simulink model "dual500MHzPFB"  (Simulink 6.2)
settings: Solver=ode45  StartTime=0.0  StopTime=10000  RelTol=1e-3
libraries: xbsIndex_r3 x2070, casper_library x180, xps_library x12, gtkWave x5, gavrt_library x1
(part 1 of 20)
settings Model: LastModifiedBy=Glenn
settings DebuggingCC: SolverPrmCheckMsg=warning

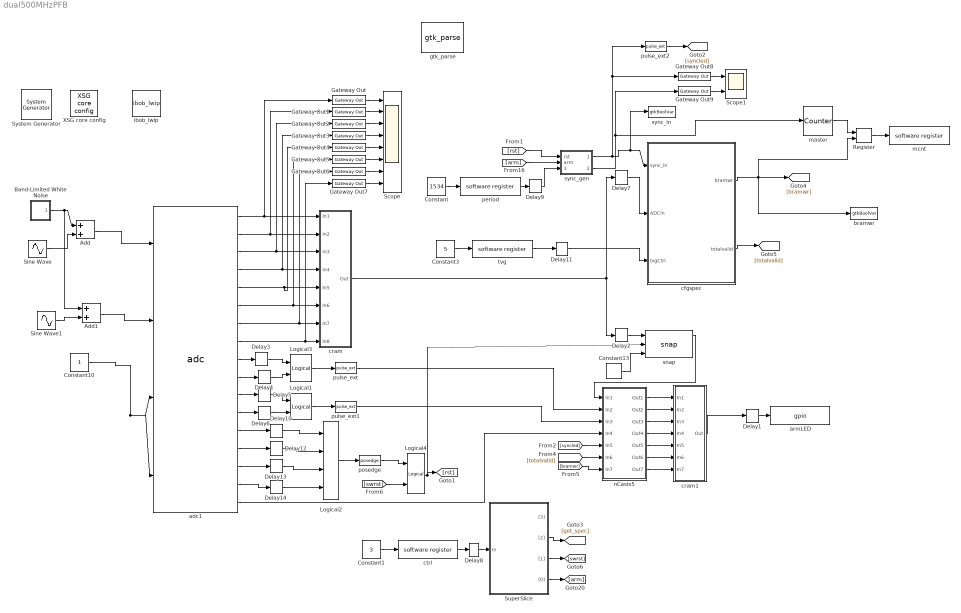
== system dual500MHzPFB ==
  " System Generator" : xbsIndex_r3/ System Generator  Tag=genX  xilinxfamily=Virtex2P  part=xc2vp50  speed=-7  package=ff1152  synthesis_tool=XST  directory=C:/casper_work/scratch/newspec/dual500MHzPFB/sysgen  testbench=off  simulink_period=1  sysclk_period=3.9063  incr_netlist=off  trim_vbits=Everywhere in SubSystem  dbl_ovrd=According to Block Masks  core_generation=According to Block Masks  run_coregen=off  deprecated_control=off  eval_field=0
      settings: AttributesFormatString=System\nGenerator
  Add : Sum  OutScaling=2^-10
  Add1 : Sum  OutScaling=2^-10
  Band-Limited White Noise : Subsystem  AncestorBlock=simulink/Sources/Band-Limited White Noise  mask(Band-Limited White Noise.){Cov=0, Ts=0.25, seed=[23341], VectorParams1D=on}
      mask prompts: Cov "Noise power:"; Ts "Sample time:"; VectorParams1D "Interpret vector parameters as 1-D"
      mask help: The Band-Limited White Noise block generates normally distributed random numbers that are suitable for use in continuous or hybrid systems.
      mask init:
      | if any(Cov < 0),
      | 	error('The ''Noise power'' must be positive. '),
      | end;
      | 
      | r = [-0.4326
      |    -1.6656
      |     0.1253
      |     0.2877
      |    -1.1465
      |     1.1909
      |     1.1892
      |    -0.0376
      |     0.3273
      |     0.1746
      |    -0.1867
      |     0.7258]';
      | 
      | r2 = [r(1),r;r,r(12)]; 
      | t =[1:13;1:13]; 
      | 
      | if any(Ts==-1), 
      | 	error('Sample time (-1) is set to be back-inherited from the block(s) it drives. You should explicitly specify the sample time of the source block. '), 
      | end;
      | set_param([gcb '/White Noise'],'VectorParams1D',VectorParams1D);
      mask Help: Implemented using white noise into Zero-Order Hold block. The seed and power can be vectors of the same length to produce a vector of white noise sources. For faster simulation, set sample time to the highest value possible but in accordance with the fastest dynamics of system.
      mask Display: plot(t(:),r2(:))
  Constant : Constant  Value=1534
  Constant1 : Constant  Value=3
  Constant10 : Constant
  Constant13 : xbsIndex_r3/Constant  const=1  equ=P=C  arith_type=Boolean  n_bits=8  bin_pt=0  opselect=C  inp2=PCIN>>17  opr=+  inp1=P  carry=CIN  iostate=0  explicit_period=on  period=1  dbl_ovrd=off
  Constant3 : Constant  Value=5
  Delay{1,3..6} (5 alike) : xbsIndex_r3/Delay  latency=4  reg_retiming=on  explicit_period=off  period=1  en=off  accept_only_valid=off  init_zero=on  dbl_ovrd=off  show_param=off
      settings: xl_area=[0, 0, 0, 0, 0, 0, 0]
  Delay{10,12..14} (4 alike) : xbsIndex_r3/Delay  latency=1  reg_retiming=on  explicit_period=off  period=1  en=off  accept_only_valid=off  init_zero=on  dbl_ovrd=off  show_param=off
      settings: xl_area=[0, 0, 0, 0, 0, 0, 0]
  Delay11 : xbsIndex_r3/Delay  latency=2  reg_retiming=on  explicit_period=off  period=1  en=off  accept_only_valid=off  init_zero=on  dbl_ovrd=off  show_param=off
      settings: xl_area=[0, 0, 0, 0, 0, 0, 0]
  Delay2 : xbsIndex_r3/Delay  latency=3  reg_retiming=on  explicit_period=off  period=1  en=off  accept_only_valid=off  init_zero=on  dbl_ovrd=off  show_param=off
      settings: xl_area=[0, 0, 0, 0, 0, 0, 0]
  Delay7 : xbsIndex_r3/Delay  latency=2  reg_retiming=on  explicit_period=off  period=1  en=off  accept_only_valid=off  init_zero=on  dbl_ovrd=off  show_param=off
      settings: xl_area=[0, 0, 0, 0, 0, 0, 0]
  Delay8 : xbsIndex_r3/Delay  latency=3  reg_retiming=on  explicit_period=off  period=1  en=off  accept_only_valid=off  init_zero=on  dbl_ovrd=off  show_param=off
      settings: xl_area=[0, 0, 0, 0, 0, 0, 0]
  Delay9 : xbsIndex_r3/Delay  latency=2  reg_retiming=on  explicit_period=off  period=1  en=off  accept_only_valid=off  init_zero=on  dbl_ovrd=off  show_param=off
      settings: xl_area=[0, 0, 0, 0, 0, 0, 0]
  Gateway Out{,1..9} (10 alike) : xbsIndex_r3/Gateway Out  output_type=Double  nbits=8  bin_pt=6  arith_type=Boolean  quantization=Truncate  overflow=Wrap  hdl_port=on  timing_constraint=None  locs_specified=off  LOCs={}  needs_fixed_name=off  show_param=off
      settings: xl_area=[0, 0, 0, 0, 0, 0, 0]
  Logical1 : xbsIndex_r3/Logical  logical_function=OR  inputs=2  precision=Full  arith_type=Unsigned  n_bits=8  bin_pt=2  align_bp=on  latency=0  explicit_period=off  period=1  en=off  dbl_ovrd=off  show_param=off
      settings: xl_area=[0, 0, 0, 0, 0, 0, 0]
  Logical2 : xbsIndex_r3/Logical  logical_function=OR  inputs=4  precision=Full  arith_type=Unsigned  n_bits=8  bin_pt=2  align_bp=on  latency=1  explicit_period=off  period=1  en=off  dbl_ovrd=off  show_param=off
      settings: xl_area=[0, 0, 0, 0, 0, 0, 0]
  Logical3 : xbsIndex_r3/Logical  logical_function=OR  inputs=2  precision=Full  arith_type=Unsigned  n_bits=8  bin_pt=2  align_bp=on  latency=0  explicit_period=off  period=1  en=off  dbl_ovrd=off  show_param=off
      settings: xl_area=[0, 0, 0, 0, 0, 0, 0]
  Logical4 : xbsIndex_r3/Logical  logical_function=OR  inputs=2  precision=Full  arith_type=Unsigned  n_bits=8  bin_pt=2  align_bp=on  latency=1  explicit_period=off  period=1  en=off  dbl_ovrd=off  show_param=off
      settings: xl_area=[0, 0, 0, 0, 0, 0, 0]
  Register : xbsIndex_r3/Register  init=0  reg_only_valid=off  explicit_period=off  period=1  rst=off  en=on  out_en=off  dbl_ovrd=off  show_param=off
      settings: xl_area=[0, 0, 0, 0, 0, 0, 0]
  Scope : Scope  NumInputPorts=8
      settings: YMin=-5~-5~-5~-5~-5~-5~-5~-5  YMax=5~5~5~5~5~5~5~5
  Scope1 : Scope  NumInputPorts=2
      settings: YMin=-5~-5  YMax=5~5  SaveName=ScopeData6
  Sine Wave : Sin  Amplitude=.1  Bias=.5  Frequency=4.1*2*pi  Samples=8  SampleTime=.25
  Sine Wave1 : Sin  Amplitude=.1  Bias=.5  Frequency=4.1*2*pi  Phase=(-pi/2)  Samples=8  SampleTime=.25  Offset=2
  SuperSlice : Subsystem  AncestorBlock=gavrt_library/SuperSlice  mask(superslice){slices=-1*ones(1,4)}
      mask prompts: slices "Slice pattern"
      mask help:
      | Slices the input word into consecutive outputs of arbitrary width.
      | Slice pattern should be a vector with each entry representing the width of that particular slice. The first entry is the MSB slice and the last is the LSB slice.
      | If a slice is given width -1, that slice will have a boolean output.
      | Ex: -1*ones(1,32)  -- Slice a 32 bit word into seperate boolean flags
      | [16, 8, -1*ones(1,8)] -- Slice a 32 bit word into the MSW, a byte, and the least significant 8 bits
      mask init:
      | superslice_init(gcb, 'slices', slices);
  XSG core config : xps_library/XSG core config  Tag=xps:xsg  hw_sys=iBOB  ibob_linux=off  clk_src=adc0_clk  gpio_clk_io_group=iBOB:sma  gpio_clk_bit_index=0  clk_rate=256  sample_period=1  synthesis_tool=XST  mpc_type=powerpc405
  adc1 : xps_library/adc  Tag=xps:adc  adc_brd=iBOB:adc0  adc_clk_rate=1024  adc_interleave=off  sample_period=1
  armLED : xps_library/gpio  Tag=xps:gpio  io_group=iBOB:led  io_dir=out  arith_type=Unsigned  bitwidth=7  bin_pt=0  bit_index=0:6  sample_period=1  use_single_ended=off  use_ddr=off  reg_iob=on  reg_clk_phase=0  termination=None
  bramwr : gtkWave/gtkBoolVar
  cfgspec : Subsystem
  cram : Subsystem  AncestorBlock=gavrt_library/cram  mask(cram){num_slice=8}
      mask prompts: num_slice "Number of slices"
      mask help: Concatenates inputs together after forcing binary point to zero.
      mask init:
      | cram_init(gcb, ...
      |     'num_slice', num_slice);
  cram1 : Subsystem  AncestorBlock=gavrt_library/cram  mask(cram){num_slice=7}
      mask prompts: num_slice "Number of slices"
      mask help: Concatenates inputs together after forcing binary point to zero.
      mask init:
      | cram_init(gcb, ...
      |     'num_slice', num_slice);
  ctrl : xps_library/software register  Tag=xps:sw_reg  io_dir=From Processor  arith_type=Unsigned  bitwidth=32  bin_pt=0  sample_period=1  gw_name=dual500MHzPFB_ctrl_user_data_out
  gtk_parse : gtkWave/gtk_parse  dummy=0
  ibob_lwip : xps_library/ibob_lwip
  master : xbsIndex_r3/Counter  cnt_type=Free Running  n_bits=32  bin_pt=0  arith_type=Unsigned  start_count=0  cnt_to=Inf  cnt_by_val=1  operation=Up  explicit_period=off  period=1  load_pin=off  rst=on  en=off  dbl_ovrd=off  show_param=off  use_rpm=on  gen_core=off
      settings: xl_area=[0, 0, 0, 0, 0, 0, 0]
  mcnt : xps_library/software register  Tag=xps:sw_reg  io_dir=To Processor  arith_type=Unsigned  bitwidth=32  bin_pt=0  sample_period=1  gw_name=dual500MHzPFB_mcnt_user_data_in
  nCasts5 : Subsystem  AncestorBlock=xaui_align_lib/XAUIdemux/nCasts5  mask(ncasts){ncasts=7, arith_type=0, nbits=1, bin_pt=0}
      mask prompts: ncasts "Number of Casts"; arith_type "Arithmetic Type (0=Unsigned, 1=Signed, 2=Boolean)"; nbits "Output Bit Width"; bin_pt "Binary Point"
      mask init:
      | ncasts_init(gcb, ...
      |     'ncasts', ncasts, ...
      |     'arith_type', arith_type, ...
      |     'nbits', nbits, ...
      |     'bin_pt', bin_pt);
  period : xps_library/software register  Tag=xps:sw_reg  io_dir=From Processor  arith_type=Unsigned  bitwidth=32  bin_pt=0  sample_period=1  gw_name=dual500MHzPFB_period_user_data_out
  posedge : casper_library/Misc/posedge  Tag=Rising Edge Detector
  pulse_ext : casper_library/Misc/pulse_ext  pulse_len=(2^23)-1
  pulse_ext1 : casper_library/Misc/pulse_ext  pulse_len=(2^23)-1
  pulse_ext2 : casper_library/Misc/pulse_ext  pulse_len=2^20
  snap : gavrt_library/snap  nsamples=11  latency=2
  sync_gen : Subsystem
  sync_in : gtkWave/gtkBoolVar
  tvg : xps_library/software register  Tag=xps:sw_reg  io_dir=From Processor  arith_type=Unsigned  bitwidth=32  bin_pt=0  sample_period=1  gw_name=dual500MHzPFB_tvg_user_data_out
  wires:
  Constant10/1 -> adc1/3, adc1/4
  cram/1(Out) -> Delay2/1, Delay7/1
  Delay2/1 -> snap/1
  Constant13/1 -> snap/3
  adc1/1 -> cram/1(In1), Gateway Out/1
  adc1/2 -> cram/2(In2), Gateway Out1/1
  adc1/3 -> cram/3(In3), Gateway Out2/1
  adc1/4 -> cram/4(In4), Gateway Out3/1
  adc1/5 -> cram/5(In5), Gateway Out4/1
  adc1/6 -> cram/6(In6), Gateway Out5/1
  adc1/7 -> cram/7(In7), Gateway Out6/1
  adc1/8 -> cram/8(In8), Gateway Out7/1
  adc1/9 -> Delay3/1
  adc1/10 -> Delay4/1
  adc1/11 -> Delay5/1
  adc1/12 -> Delay6/1
  Logical3/1 -> pulse_ext/1
  Logical1/1 -> pulse_ext1/1
  nCasts5/1(Out1) -> cram1/1(In1)
  nCasts5/2(Out2) -> cram1/2(In2)
  nCasts5/3(Out3) -> cram1/3(In3)
  cram1/1(Out) -> Delay1/1
  Delay1/1 -> armLED/1
  Delay3/1 -> Logical3/1
  Delay4/1 -> Logical3/2
  Delay5/1 -> Logical1/1
  Delay6/1 -> Logical1/2
  nCasts5/4(Out4) -> cram1/4(In4)
  pulse_ext/1 -> nCasts5/2(In2)
  pulse_ext1/1 -> nCasts5/3(In3)
  adc1/17 -> nCasts5/4(In4)
  Gateway Out/1 -> Scope/1
  Gateway Out1/1 -> Scope/2
  Gateway Out2/1 -> Scope/3
  Gateway Out3/1 -> Scope/4
  Gateway Out4/1 -> Scope/5
  Gateway Out5/1 -> Scope/6
  Gateway Out6/1 -> Scope/7
  Gateway Out7/1 -> Scope/8
  sync_gen/1(sync) -> pulse_ext2/1, Gateway Out8/1, cfgspec/1(sync_in), sync_in/1
  Band-Limited White Noise/1(Out1) -> Add/1, Add1/1
  Sine Wave/1 -> Add/2
  Add/1 -> adc1/1
  Sine Wave1/1 -> Add1/2
  Add1/1 -> adc1/2
  Constant/1 -> period/1
  period/1 -> Delay9/1
  Constant1/1 -> ctrl/1
  ctrl/1 -> Delay8/1
  SuperSlice/4("[0]") -> [arm]
  [arm] -> sync_gen/2(arm)
  [rst] -> sync_gen/1(rst)
  pulse_ext2/1 -> [syncled]
  nCasts5/5(Out5) -> cram1/5(In5)
  [syncled] -> nCasts5/5(In5)
  Gateway Out8/1 -> Scope1/1
  Gateway Out9/1 -> Scope1/2
  sync_gen/2(mrst) -> Gateway Out9/1, master/1
  snap/1 -> nCasts5/1(In1)
  SuperSlice/2("[2]") -> [get_spec]
  nCasts5/6(Out6) -> cram1/6(In6)
  nCasts5/7(Out7) -> cram1/7(In7)
  [totalvalid] -> nCasts5/6(In6)
  [bramwr] -> nCasts5/7(In7)
  cfgspec/2(totalvalid) -> [totalvalid]
  Delay7/1 -> cfgspec/2(ADCin)
  Delay8/1 -> SuperSlice/1(In)
  Delay9/1 -> sync_gen/3(period)
  Logical2/1 -> posedge/1
  adc1/13 -> Delay10/1
  adc1/14 -> Delay12/1
  adc1/15 -> Delay13/1
  adc1/16 -> Delay14/1
  SuperSlice/3("[1]") -> [swrst]
  posedge/1 -> Logical4/1
  [swrst] -> Logical4/2
  Logical4/1 -> [rst], snap/2
  cfgspec/1(bramwr) -> [bramwr], bramwr/1, Register/2
  master/1 -> Register/1
  Register/1 -> mcnt/1
  tvg/1 -> Delay11/1
  Constant3/1 -> tvg/1
  Delay11/1 -> cfgspec/3(tvgCtrl)
  Delay10/1 -> Logical2/1
  Delay12/1 -> Logical2/2
  Delay13/1 -> Logical2/3
  Delay14/1 -> Logical2/4

== system dual500MHzPFB/Band-Limited White Noise ==
  Output : Gain  Gain=[sqrt(Cov)]/[sqrt(Ts)]  SaturateOnIntegerOverflow=on
  White Noise : RandomNumber  DisableCoverage=on  Seed=seed  SampleTime=Ts
  Out1 : Outport
  wires:
  Output/1 -> Out1/1
  White Noise/1 -> Output/1

== system dual500MHzPFB/SuperSlice ==
  In : Inport  Port=1  LatchInput=off
  Slice1 : xbsIndex_r3/Slice  mode=Lower Bit Location + Width  nbits=1  bit1=-3  base1=MSB of Input  bit0=3  base0=LSB of Input  boolean_output=on  explicit_period=off  period=1  dbl_ovrd=off
  Slice2 : xbsIndex_r3/Slice  mode=Lower Bit Location + Width  nbits=1  bit1=-2  base1=MSB of Input  bit0=2  base0=LSB of Input  boolean_output=on  explicit_period=off  period=1  dbl_ovrd=off
  Slice3 : xbsIndex_r3/Slice  mode=Lower Bit Location + Width  nbits=1  bit1=-1  base1=MSB of Input  bit0=1  base0=LSB of Input  boolean_output=on  explicit_period=off  period=1  dbl_ovrd=off
  Slice4 : xbsIndex_r3/Slice  mode=Lower Bit Location + Width  nbits=1  bit1=0  base1=MSB of Input  bit0=0  base0=LSB of Input  boolean_output=on  explicit_period=off  period=1  dbl_ovrd=off
  "[3]" : Outport
  "[2]" : Outport  Port=2
  "[1]" : Outport  Port=3
  "[0]" : Outport  Port=4
  wires:
  In/1 -> Slice4/1, Slice3/1, Slice2/1, Slice1/1
  Slice1/1 -> "[3]"/1
  Slice2/1 -> "[2]"/1
  Slice3/1 -> "[1]"/1
  Slice4/1 -> "[0]"/1

== system dual500MHzPFB/cfgspec ==
  sync_in : Inport  Port=1  LatchInput=off
  ADCin : Inport  Port=2  LatchInput=off
  tvgCtrl : Inport  Port=3  LatchInput=off
  Counter : xbsIndex_r3/Counter  cnt_type=Free Running  n_bits=8  bin_pt=0  arith_type=Unsigned  start_count=0  cnt_to=Inf  cnt_by_val=1  operation=Up  explicit_period=off  period=1  load_pin=on  rst=on  en=on  dbl_ovrd=off  show_param=off  use_rpm=on  gen_core=off
      settings: xl_area=[0, 0, 0, 0, 0, 0, 0]
  Delay{1..4,6..7} (6 alike) : xbsIndex_r3/Delay  latency=2  reg_retiming=off  explicit_period=off  period=1  en=off  accept_only_valid=off  init_zero=on  dbl_ovrd=off  show_param=off
      settings: xl_area=[0, 0, 0, 0, 0, 0, 0]
  Delay5 : xbsIndex_r3/Delay  latency=1  reg_retiming=off  explicit_period=off  period=1  en=off  accept_only_valid=off  init_zero=on  dbl_ovrd=off  show_param=off
      settings: xl_area=[0, 0, 0, 0, 0, 0, 0]
  Delay9 : xbsIndex_r3/Delay  latency=7  reg_retiming=off  explicit_period=off  period=1  en=off  accept_only_valid=off  init_zero=on  dbl_ovrd=off  show_param=off
      settings: xl_area=[0, 0, 0, 0, 0, 0, 0]
  FFT_Subsystem : Subsystem
  Inverter : xbsIndex_r3/Inverter  latency=0  explicit_period=off  period=1  en=off  dbl_ovrd=off  show_param=off
      settings: xl_area=[0, 0, 0, 0, 0, 0, 0]
  Logical : xbsIndex_r3/Logical  logical_function=AND  inputs=2  precision=Full  arith_type=Unsigned  n_bits=8  bin_pt=2  align_bp=on  latency=0  explicit_period=off  period=1  en=off  dbl_ovrd=off  show_param=off
      settings: xl_area=[0, 0, 0, 0, 0, 0, 0]
  Mux : xbsIndex_r3/Mux  inputs=2  precision=Full  arith_type="Signed  (2's comp)"  n_bits=8  bin_pt=2  quantization=Truncate  overflow=Wrap  latency=2  explicit_period=off  period=1  en=off  dbl_ovrd=off  show_param=off  mux_type=off  use_rpm=off  gen_core=off
      settings: xl_area=[0, 0, 0, 0, 0, 0, 0]
  Negate : xbsIndex_r3/Negate  precision=User Defined  arith_type="Signed  (2's comp)"  n_bits=8  bin_pt=7  quantization=Truncate  overflow=Wrap  latency=0  explicit_period=off  period=1  en=off  dbl_ovrd=off  use_core=on  show_param=on  use_rpm=on  gen_core=off
      settings: xl_area=[0, 0, 0, 0, 0, 0, 0]
  Negate1 : xbsIndex_r3/Negate  precision=User Defined  arith_type="Signed  (2's comp)"  n_bits=8  bin_pt=7  quantization=Truncate  overflow=Wrap  latency=0  explicit_period=off  period=1  en=off  dbl_ovrd=off  use_core=on  show_param=on  use_rpm=on  gen_core=off
      settings: xl_area=[0, 0, 0, 0, 0, 0, 0]
  PFB_Subsystem : Subsystem
  Reinterpret : xbsIndex_r3/Reinterpret  force_arith_type=on  arith_type="Signed  (2's comp)"  force_bin_pt=on  bin_pt=7  force_valid=on
  SuperSlice : Subsystem  AncestorBlock=gavrt_library/SuperSlice  mask(superslice){slices=[16 8 -1*ones(1,8)]}
      mask prompts: slices "Slice pattern"
      mask help:
      | Slices the input word into consecutive outputs of arbitrary width.
      | Slice pattern should be a vector with each entry representing the width of that particular slice. The first entry is the MSB slice and the last is the LSB slice.
      | If a slice is given width -1, that slice will have a boolean output.
      | Ex: -1*ones(1,32)  -- Slice a 32 bit word into seperate boolean flags
      | [16, 8, -1*ones(1,8)] -- Slice a 32 bit word into the MSW, a byte, and the least significant 8 bits
      mask init:
      | superslice_init(gcb, 'slices', slices);
  cram : Subsystem  AncestorBlock=gavrt_library/cram  mask(cram){num_slice=4}
      mask prompts: num_slice "Number of slices"
      mask help: Concatenates inputs together after forcing binary point to zero.
      mask init:
      | cram_init(gcb, ...
      |     'num_slice', num_slice);
  cram1 : Subsystem  AncestorBlock=gavrt_library/cram  mask(cram){num_slice=8}
      mask prompts: num_slice "Number of slices"
      mask help: Concatenates inputs together after forcing binary point to zero.
      mask init:
      | cram_init(gcb, ...
      |     'num_slice', num_slice);
  nCasts1 : Subsystem  AncestorBlock=gavrt_library/nCasts  mask(ncasts){ncasts=4, arith_type=0, nbits=32, bin_pt=31}
      mask prompts: ncasts "Number of Casts"; arith_type "Arithmetic Type (0=Unsigned, 1=Signed, 2=Boolean)"; nbits "Output Bit Width"; bin_pt "Binary Point"
      mask init:
      | ncasts_init(gcb, ...
      |     'ncasts', ncasts, ...
      |     'arith_type', arith_type, ...
      |     'nbits', nbits, ...
      |     'bin_pt', bin_pt);
  power : Subsystem  mask{BitWidth=18, mult_latency=3, add_latency=4}
      mask prompts: BitWidth "Bit Width"; mult_latency "Multiplier Latency"; add_latency "Add Latency"
  power1 : Subsystem  mask{BitWidth=18, mult_latency=3, add_latency=4}
      mask prompts: BitWidth "Bit Width"; mult_latency "Multiplier Latency"; add_latency "Add Latency"
  power2 : Subsystem  mask{BitWidth=18, mult_latency=3, add_latency=4}
      mask prompts: BitWidth "Bit Width"; mult_latency "Multiplier Latency"; add_latency "Add Latency"
  power3 : Subsystem  mask{BitWidth=18, mult_latency=3, add_latency=4}
      mask prompts: BitWidth "Bit Width"; mult_latency "Multiplier Latency"; add_latency "Add Latency"
  uncram : Subsystem  AncestorBlock=gavrt_library/uncram  mask(uncram){num_slice=4, slice_width=36, bin_pt=0, arith_type=0}
      mask prompts: num_slice "Number of slices"; slice_width "Slice Width"; bin_pt "Output Binary Point"; arith_type "Output Arithmetic Type (0=Unsigned, 1=Signed)"
      mask help: Takes a concatenated input and slices it up into even pieces and reinterprets them as signed fixed point numbers with a given binary point.
      mask init:
      | uncram_init(gcb, ...
      |     'num_slice', num_slice, ...
      |     'slice_width', slice_width, ...
      |     'bin_pt', bin_pt, ...
      |     'arith_type', arith_type);
      settings: AttributesFormatString=UFix_36_0
  vacc : Subsystem
  bramwr : Outport
  totalvalid : Outport  Port=2
  wires:
  nCasts1/1(Out1) -> cram/1(In1)
  nCasts1/2(Out2) -> cram/2(In2)
  nCasts1/3(Out3) -> cram/3(In3)
  nCasts1/4(Out4) -> cram/4(In4)
  cram/1(Out) -> vacc/2(din)
  Delay9/1 -> vacc/1(sync)
  vacc/1(bramwr) -> bramwr/1
  vacc/2(totalvalid) -> totalvalid/1
  sync_in/1 -> Logical/1, Delay5/1
  FFT_Subsystem/1(syncOut1) -> [sync0], Delay4/1
  FFT_Subsystem/3(dataOut) -> uncram/1(In)
  uncram/1(Out1) -> Delay6/1
  uncram/2(Out2) -> Delay7/1
  uncram/3(Out3) -> Delay2/1
  uncram/4(Out4) -> Delay3/1
  Delay6/1 -> power/1(c)
  Delay7/1 -> power1/1(c)
  Delay2/1 -> power2/1(c)
  Delay3/1 -> power3/1(c)
  power/1(power) -> nCasts1/1(In1)
  power1/1(power) -> nCasts1/2(In2)
  power2/1(power) -> nCasts1/3(In3)
  power3/1(power) -> nCasts1/4(In4)
  Delay4/1 -> Delay9/1
  Counter/1 -> Reinterpret/1
  cram1/1(Out) -> Mux/3
  ADCin/1 -> Mux/2
  Mux/1 -> PFB_Subsystem/2(dataIn)
  tvgCtrl/1 -> SuperSlice/1(In)
  Reinterpret/1 -> cram1/1(In1), cram1/2(In2), cram1/3(In3), cram1/5(In5), cram1/6(In6), cram1/7(In7), Negate1/1, Negate/1
  Negate/1 -> cram1/4(In4)
  Negate1/1 -> cram1/8(In8)
  Logical/1 -> Counter/3
  [tvgen] -> Mux/1
  [cntrst] -> Logical/2
  PFB_Subsystem/1(syncOut1) -> FFT_Subsystem/1(syncIn1)
  PFB_Subsystem/2(syncOut2) -> FFT_Subsystem/2(syncIn2)
  PFB_Subsystem/3(dataOut) -> FFT_Subsystem/3(dataIn)
  SuperSlice/1("[31:16]") -> Inverter/1
  SuperSlice/2("[15:8]") -> Counter/2
  SuperSlice/10("[0]") -> Counter/4
  SuperSlice/9("[1]") -> [cntrst]
  SuperSlice/8("[2]") -> [tvgen]
  SuperSlice/7("[3]") -> Counter/1
  Delay1/1 -> PFB_Subsystem/1(syncIn)
  Delay5/1 -> Delay1/1
  [shift] -> FFT_Subsystem/4(shift)
  Inverter/1 -> [shift]

== system dual500MHzPFB/cram ==
  In1 : Inport  Port=1  LatchInput=off
  In2 : Inport  Port=2  LatchInput=off
  In3 : Inport  Port=3  LatchInput=off
  In4 : Inport  Port=4  LatchInput=off
  In5 : Inport  Port=5  LatchInput=off
  In6 : Inport  Port=6  LatchInput=off
  In7 : Inport  Port=7  LatchInput=off
  In8 : Inport  Port=8  LatchInput=off
  Concat : S-Function  AncestorBlock=xbsIndex_r3/Concat  FunctionName=xlconcat  Parameters=sfcn_mwsv__  mask(Xilinx Bus Concatenator){num_inputs=8, explicit_period=off, period=1, dbl_ovrd=off}
      mask prompts: num_inputs "Number of Inputs"; explicit_period "Use Explicit Sample Period"; period "Sample Period  (use -1 to inherit first known input period)"; dbl_ovrd "Override with Doubles"
      mask help: Concatenates two or more inputs. Inputs must be unsigned with binary point at zero.
      mask init:
      | [designRoot, family, part, speed, package, simulinkPeriod, sysclkPeriod, dbl_ovrd, trimVbit] = xlSysgenSettings(gcb,1,1);
      | [bg,fg] = xlcmap('XBlock',dbl_ovrd);
      | iPos = get_param(gcb,'Position');
      | iWidth=iPos(3)-iPos(1); iHeight=iPos(4)-iPos(2);
      | iCx=iWidth/2;
      | iCy=iHeight/2;
      | [logoX, logoY] = xlogo(iPos);
      | 
      | 
      | 
      | 
      | % one time added for param list
      | numInputs = num_inputs + 1;
      | precision0 = 1;
      | latency = 0;
      | dblOvrd = dbl_ovrd;
      | explicitClk = explicit_period;
      | 
      | 
      | % just pass everything to s-function
      | sfcn_mwsv__ = get_param(gcb, 'MaskWSVariables');
      mask Help: eval('xlWeb(xlhtmldoclink(''Concat''))');
      mask StyleString: popup(2|3|4|5|6|7|8|9|10|11|12|13|14|15|16),checkbox,edit,checkbox
      mask CallbackString: |xlMagicCallback||
      mask Display:
      | patch([0 iWidth iWidth 0],[0 0 iHeight iHeight] , bg);
      | patch(logoX,logoY, fg);
      | port_label('input',1,'hi');
      | port_label('input',num_inputs+1,'lo');
      | port_label('output',1,'cat');
      | ;plot([0 0 iWidth iWidth 0], [0 iHeight iHeight 0 0]);
  Reinterp{1..8} (8 alike) : xbsIndex_r3/Reinterpret  force_arith_type=on  arith_type=Unsigned  force_bin_pt=on  bin_pt=0  force_valid=on
  Out : Outport
  wires:
  Concat/1 -> Out/1
  In1/1 -> Reinterp1/1
  Reinterp1/1 -> Concat/1
  In2/1 -> Reinterp2/1
  Reinterp2/1 -> Concat/2
  In3/1 -> Reinterp3/1
  Reinterp3/1 -> Concat/3
  In4/1 -> Reinterp4/1
  Reinterp4/1 -> Concat/4
  In5/1 -> Reinterp5/1
  Reinterp5/1 -> Concat/5
  In6/1 -> Reinterp6/1
  Reinterp6/1 -> Concat/6
  In7/1 -> Reinterp7/1
  Reinterp7/1 -> Concat/7
  In8/1 -> Reinterp8/1
  Reinterp8/1 -> Concat/8

== system dual500MHzPFB/cram1 ==
  In1 : Inport  Port=1  LatchInput=off
  In2 : Inport  Port=2  LatchInput=off
  In3 : Inport  Port=3  LatchInput=off
  In4 : Inport  Port=4  LatchInput=off
  In5 : Inport  Port=5  LatchInput=off
  In6 : Inport  Port=6  LatchInput=off
  In7 : Inport  Port=7  LatchInput=off
  Concat : S-Function  AncestorBlock=xbsIndex_r3/Concat  FunctionName=xlconcat  Parameters=sfcn_mwsv__  mask(Xilinx Bus Concatenator){num_inputs=7, explicit_period=off, period=1, dbl_ovrd=off}
      mask prompts: num_inputs "Number of Inputs"; explicit_period "Use Explicit Sample Period"; period "Sample Period  (use -1 to inherit first known input period)"; dbl_ovrd "Override with Doubles"
      mask help: Concatenates two or more inputs. Inputs must be unsigned with binary point at zero.
      mask init: same as dual500MHzPFB/cram/Concat
      mask Help: eval('xlWeb(xlhtmldoclink(''Concat''))');
      mask StyleString: popup(2|3|4|5|6|7|8|9|10|11|12|13|14|15|16),checkbox,edit,checkbox
      mask CallbackString: |xlMagicCallback||
      mask Display:
      | patch([0 iWidth iWidth 0],[0 0 iHeight iHeight] , bg);
      | patch(logoX,logoY, fg);
      | port_label('input',1,'hi');
      | port_label('input',num_inputs+1,'lo');
      | port_label('output',1,'cat');
      | ;plot([0 0 iWidth iWidth 0], [0 iHeight iHeight 0 0]);
  Reinterp{1..7} (7 alike) : xbsIndex_r3/Reinterpret  force_arith_type=on  arith_type=Unsigned  force_bin_pt=on  bin_pt=0  force_valid=on
  Out : Outport
  wires:
  Concat/1 -> Out/1
  In1/1 -> Reinterp1/1
  Reinterp1/1 -> Concat/1
  In2/1 -> Reinterp2/1
  Reinterp2/1 -> Concat/2
  In3/1 -> Reinterp3/1
  Reinterp3/1 -> Concat/3
  In4/1 -> Reinterp4/1
  Reinterp4/1 -> Concat/4
  In5/1 -> Reinterp5/1
  Reinterp5/1 -> Concat/5
  In6/1 -> Reinterp6/1
  Reinterp6/1 -> Concat/6
  In7/1 -> Reinterp7/1
  Reinterp7/1 -> Concat/7

== system dual500MHzPFB/nCasts5 ==
  In1 : Inport  Port=1  LatchInput=off
  In2 : Inport  Port=2  LatchInput=off
  In3 : Inport  Port=3  LatchInput=off
  In4 : Inport  Port=4  LatchInput=off
  In5 : Inport  Port=5  LatchInput=off
  In6 : Inport  Port=6  LatchInput=off
  In7 : Inport  Port=7  LatchInput=off
  Cast{1..7} (7 alike) : xbsIndex_r3/Convert  arith_type=Unsigned  n_bits=1  bin_pt=0  quantization=Truncate  overflow=Wrap  latency=0  explicit_period=off  period=1  dbl_ovrd=off  show_param=off  inserted_by_tool=off  pipeline=off
      settings: xl_area=[0, 0, 0, 0, 0, 0, 0]
  Out1 : Outport
  Out2 : Outport  Port=2
  Out3 : Outport  Port=3
  Out4 : Outport  Port=4
  Out5 : Outport  Port=5
  Out6 : Outport  Port=6
  Out7 : Outport  Port=7
  wires:
  In1/1 -> Cast1/1
  Cast1/1 -> Out1/1
  In2/1 -> Cast2/1
  Cast2/1 -> Out2/1
  In3/1 -> Cast3/1
  Cast3/1 -> Out3/1
  In4/1 -> Cast4/1
  Cast4/1 -> Out4/1
  In5/1 -> Cast5/1
  Cast5/1 -> Out5/1
  In6/1 -> Cast6/1
  Cast6/1 -> Out6/1
  In7/1 -> Cast7/1
  Cast7/1 -> Out7/1

== system dual500MHzPFB/sync_gen ==
  note: mrst must be correctly aligned with a sync pulse
  rst : Inport  Port=1  LatchInput=off
  arm : Inport  Port=2  LatchInput=off
  period : Inport  Port=3  LatchInput=off
  Constant1 : xbsIndex_r3/Constant  const=1  equ=P=C  arith_type=Boolean  n_bits=1  bin_pt=0  opselect=C  inp2=PCIN>>17  opr=+  inp1=P  carry=CIN  iostate=0  explicit_period=on  period=1  dbl_ovrd=off
  Constant10 : xbsIndex_r3/Constant  const=1  equ=P=C  arith_type=Boolean  n_bits=1  bin_pt=0  opselect=C  inp2=PCIN>>17  opr=+  inp1=P  carry=CIN  iostate=0  explicit_period=on  period=1  dbl_ovrd=off
  Convert : xbsIndex_r3/Convert  arith_type=Boolean  n_bits=8  bin_pt=6  quantization=Truncate  overflow=Wrap  latency=0  explicit_period=off  period=1  dbl_ovrd=off  show_param=off  inserted_by_tool=off  pipeline=off
      settings: xl_area=[0, 0, 0, 0, 0, 0, 0]
  Counter1 : xbsIndex_r3/Counter  cnt_type=Free Running  n_bits=24  bin_pt=0  arith_type=Unsigned  start_count=1  cnt_to=Inf  cnt_by_val=1  operation=Up  explicit_period=on  period=1  load_pin=off  rst=on  en=off  dbl_ovrd=off  show_param=off  use_rpm=on  gen_core=off
      settings: xl_area=[0, 0, 0, 0, 0, 0, 0]
  Logical : xbsIndex_r3/Logical  logical_function=OR  inputs=2  precision=Full  arith_type=Unsigned  n_bits=8  bin_pt=2  align_bp=on  latency=0  explicit_period=off  period=1  en=off  dbl_ovrd=off  show_param=off
      settings: xl_area=[0, 0, 0, 0, 0, 0, 0]
  Logical1 : xbsIndex_r3/Logical  logical_function=AND  inputs=2  precision=Full  arith_type=Unsigned  n_bits=8  bin_pt=2  align_bp=on  latency=0  explicit_period=off  period=1  en=off  dbl_ovrd=off  show_param=off
      settings: xl_area=[0, 0, 0, 0, 0, 0, 0]
  Register : xbsIndex_r3/Register  init=0  reg_only_valid=off  explicit_period=off  period=1  rst=on  en=on  out_en=off  dbl_ovrd=off  show_param=off
      settings: xl_area=[0, 0, 0, 0, 0, 0, 0]
  Register2 : xbsIndex_r3/Register  init=0  reg_only_valid=off  explicit_period=off  period=1  rst=on  en=on  out_en=off  dbl_ovrd=off  show_param=off
      settings: xl_area=[0, 0, 0, 0, 0, 0, 0]
  Relational : xbsIndex_r3/Relational  mode=a>=b  latency=2  explicit_period=off  period=1  en=off  dbl_ovrd=off  show_param=off
      settings: xl_area=[0, 0, 0, 0, 0, 0, 0]
  posedge1 : Subsystem  Tag=Rising Edge Detector
  posedge2 : Subsystem  Tag=Rising Edge Detector
  posedge3 : Subsystem  Tag=Rising Edge Detector
  posedge4 : Subsystem  Tag=Rising Edge Detector
  sync : Outport
  mrst : Outport  Port=2
  wires:
  Register/1 -> posedge1/1(In)
  Constant10/1 -> Register/1
  posedge2/1(Out) -> Register/2, Register2/2
  arm/1 -> posedge2/1(In)
  rst/1 -> Register/3, Register2/3
  Counter1/1 -> Relational/1
  Relational/1 -> Convert/1
  period/1 -> Relational/2
  Convert/1 -> posedge4/1(In)
  posedge1/1(Out) -> Logical/1
  Logical/1 -> Counter1/1
  Register2/1 -> posedge3/1(In)
  Constant1/1 -> Register2/1
  posedge3/1(Out) -> Logical1/2
  Logical1/1 -> mrst/1
  posedge4/1(Out) -> sync/1, Logical/2, Logical1/1

== system dual500MHzPFB/cfgspec/FFT_Subsystem ==
  syncIn1 : Inport  Port=1  LatchInput=off
  syncIn2 : Inport  Port=2  LatchInput=off
  dataIn : Inport  Port=3  LatchInput=off
  shift : Inport  Port=4  LatchInput=off
  cram : Subsystem  AncestorBlock=gavrt_library/cram  mask(cram){num_slice=4}
      mask prompts: num_slice "Number of slices"
      mask help: Concatenates inputs together after forcing binary point to zero.
      mask init:
      | cram_init(gcb, ...
      |     'num_slice', num_slice);
  fft_wideband_real : Subsystem  AncestorBlock=casper_library/FFTs/fft_wideband_real  mask(fft_wideband_real){FFTSize=10, BitWidth=18, n_inputs=2, quantization=Truncate, overflow=Wrap, add_latency=3, mult_latency=3, bram_latency=2}
      mask prompts: FFTSize "Size of FFT: (2^?)"; BitWidth "Bit Width"; n_inputs "Number of Simultaneous Inputs: (2^?)"; quantization "Quantization Behavior"; overflow "Overflow Behavior"; add_latency "Add Latency"; mult_latency "Mult Latency"; bram_latency "BRAM Latency"
      mask init:
      | fft_wideband_real_init(gcb,...
      |     'FFTSize', FFTSize,...
      |     'BitWidth', BitWidth,...
      |     'n_inputs', n_inputs,...
      |     'quantization', quantization,...
      |     'overflow', overflow,...
      |     'add_latency', add_latency,...
      |     'mult_latency', mult_latency,...
      |     'bram_latency', bram_latency);
      settings: AttributesFormatString=FFTSize=10, n_inputs=2
      mask StyleString: edit,edit,edit,popup(Truncate|Round  (unbiased: +/- Inf)|Round  (unbiased: Even Values)),popup(Wrap|Saturate|Error),edit,edit,edit
  fft_wideband_real1 : Subsystem  AncestorBlock=casper_library/FFTs/fft_wideband_real  mask(fft_wideband_real){FFTSize=10, BitWidth=18, n_inputs=2, quantization=Truncate, overflow=Wrap, add_latency=3, mult_latency=3, bram_latency=2}
      mask prompts: FFTSize "Size of FFT: (2^?)"; BitWidth "Bit Width"; n_inputs "Number of Simultaneous Inputs: (2^?)"; quantization "Quantization Behavior"; overflow "Overflow Behavior"; add_latency "Add Latency"; mult_latency "Mult Latency"; bram_latency "BRAM Latency"
      mask init: same as dual500MHzPFB/cfgspec/FFT_Subsystem/fft_wideband_real
      settings: AttributesFormatString=FFTSize=10, n_inputs=2
      mask StyleString: edit,edit,edit,popup(Truncate|Round  (unbiased: +/- Inf)|Round  (unbiased: Even Values)),popup(Wrap|Saturate|Error),edit,edit,edit
  uncram : Subsystem  AncestorBlock=gavrt_library/uncram  mask(uncram){num_slice=8, slice_width=18, bin_pt=17, arith_type=1}
      mask prompts: num_slice "Number of slices"; slice_width "Slice Width"; bin_pt "Output Binary Point"; arith_type "Output Arithmetic Type (0=Unsigned, 1=Signed)"
      mask help: Takes a concatenated input and slices it up into even pieces and reinterprets them as signed fixed point numbers with a given binary point.
      mask init:
      | uncram_init(gcb, ...
      |     'num_slice', num_slice, ...
      |     'slice_width', slice_width, ...
      |     'bin_pt', bin_pt, ...
      |     'arith_type', arith_type);
      settings: AttributesFormatString=Fix_18_17
  syncOut1 : Outport
  syncOut2 : Outport  Port=2
  dataOut : Outport  Port=3
  wires:
  shift/1 -> fft_wideband_real/2(shift), fft_wideband_real1/2(shift)
  uncram/1(Out1) -> fft_wideband_real/3(in0)
  uncram/2(Out2) -> fft_wideband_real/4(in1)
  uncram/3(Out3) -> fft_wideband_real/5(in2)
  uncram/4(Out4) -> fft_wideband_real/6(in3)
  uncram/5(Out5) -> fft_wideband_real1/3(in0)
  uncram/6(Out6) -> fft_wideband_real1/4(in1)
  uncram/7(Out7) -> fft_wideband_real1/5(in2)
  uncram/8(Out8) -> fft_wideband_real1/6(in3)
  syncIn1/1 -> fft_wideband_real/1(sync)
  fft_wideband_real/1(sync_out) -> syncOut1/1
  dataIn/1 -> uncram/1(In)
  syncIn2/1 -> fft_wideband_real1/1(sync)
  fft_wideband_real1/1(sync_out) -> syncOut2/1
  fft_wideband_real/2(out0) -> cram/1(In1)
  fft_wideband_real/3(out1) -> cram/2(In2)
  fft_wideband_real1/2(out0) -> cram/3(In3)
  fft_wideband_real1/3(out1) -> cram/4(In4)
  cram/1(Out) -> dataOut/1

== system dual500MHzPFB/cfgspec/PFB_Subsystem ==
  syncIn : Inport  Orientation=down  Port=1  LatchInput=off
  dataIn : Inport  Port=2  LatchInput=off
  cram : Subsystem  AncestorBlock=gavrt_library/cram  mask(cram){num_slice=8}
      mask prompts: num_slice "Number of slices"
      mask help: Concatenates inputs together after forcing binary point to zero.
      mask init:
      | cram_init(gcb, ...
      |     'num_slice', num_slice);
  pfb_fir_real : Subsystem  AncestorBlock=casper_library/PFBs/pfb_fir_real  mask(pfb_fir_real){PFBSize=10, TotalTaps=2, WindowType=hamming, n_inputs=2, MakeBiplex=0, BitWidthIn=8, BitWidthOut=18, CoeffBitWidth=8, CoeffDistMem=0, add_latency=2, mult_latency=2, bram_latency=2, quantization=Truncate, fwidth=1}
      mask prompts: PFBSize "Size of PFB: (2^? pnts)"; TotalTaps "Total Number of Taps:"; WindowType "Windowing Function:"; n_inputs "Number of Simultaneous Inputs: (2^?)"; MakeBiplex "Make Biplex"; BitWidthIn "Input Bitwidth:"; BitWidthOut "Output Bitwidth:"; CoeffBitWidth "Coefficient Bitwidth:"; CoeffDistMem "Use Distributed Memory for Coeffs"; add_latency "Add Latency"; mult_latency "Mult Latency"; bram_latency "BRAM Latency"; quantization "Quantization Behavior"; fwidth "Bin Width Scaling (normal=1)"
      mask init:
      | pfb_fir_real_init(gcb,...
      |     'PFBSize', PFBSize,...
      |     'TotalTaps', TotalTaps,...
      |     'WindowType', WindowType,...
      |     'n_inputs', n_inputs,...
      |     'MakeBiplex', MakeBiplex,...
      |     'BitWidthIn', BitWidthIn,...
      |     'BitWidthOut', BitWidthOut,...
      |     'CoeffBitWidth', CoeffBitWidth,...
      |     'CoeffDistMem', CoeffDistMem,...
      |     'add_latency', add_latency,...
      |     'mult_latency', mult_latency,...
      |     'bram_latency', bram_latency,...
      |     'quantization', quantization,...
      |     'fwidth', fwidth);
      settings: AttributesFormatString=taps=2, add_latency=2
      mask StyleString: edit,edit,popup(bartlett|barthannwin|blackman|blackmanharris|bohamwin|chebwin|flattopwin|gausswin|hamming|hann|kaiser|nuttallwin|parzenwin|rectwin|tukeywin|triang),edit,edit,edit,edit,edit,edit,edit,edit,edit,popup(Truncate|Round  (unbiased: +/- Inf)|Round  (unbiased: Even Values)),edit
  pfb_fir_real1 : Subsystem  AncestorBlock=casper_library/PFBs/pfb_fir_real  mask(pfb_fir_real){PFBSize=10, TotalTaps=2, WindowType=hamming, n_inputs=2, MakeBiplex=0, BitWidthIn=8, BitWidthOut=18, CoeffBitWidth=8, CoeffDistMem=0, add_latency=2, mult_latency=2, bram_latency=2, quantization=Truncate, fwidth=1}
      mask prompts: PFBSize "Size of PFB: (2^? pnts)"; TotalTaps "Total Number of Taps:"; WindowType "Windowing Function:"; n_inputs "Number of Simultaneous Inputs: (2^?)"; MakeBiplex "Make Biplex"; BitWidthIn "Input Bitwidth:"; BitWidthOut "Output Bitwidth:"; CoeffBitWidth "Coefficient Bitwidth:"; CoeffDistMem "Use Distributed Memory for Coeffs"; add_latency "Add Latency"; mult_latency "Mult Latency"; bram_latency "BRAM Latency"; quantization "Quantization Behavior"; fwidth "Bin Width Scaling (normal=1)"
      mask init: same as dual500MHzPFB/cfgspec/PFB_Subsystem/pfb_fir_real
      settings: AttributesFormatString=taps=2, add_latency=2
      mask StyleString: edit,edit,popup(bartlett|barthannwin|blackman|blackmanharris|bohamwin|chebwin|flattopwin|gausswin|hamming|hann|kaiser|nuttallwin|parzenwin|rectwin|tukeywin|triang),edit,edit,edit,edit,edit,edit,edit,edit,edit,popup(Truncate|Round  (unbiased: +/- Inf)|Round  (unbiased: Even Values)),edit
  uncram : Subsystem  AncestorBlock=gavrt_library/uncram  mask(uncram){num_slice=8, slice_width=8, bin_pt=7, arith_type=1}
      mask prompts: num_slice "Number of slices"; slice_width "Slice Width"; bin_pt "Output Binary Point"; arith_type "Output Arithmetic Type (0=Unsigned, 1=Signed, 2=Boolean)"
      mask help: Takes a concatenated input and slices it up into even pieces and reinterprets them as signed fixed point numbers with a given binary point.
      mask init:
      | uncram_init(gcb, ...
      |     'num_slice', num_slice, ...
      |     'slice_width', slice_width, ...
      |     'bin_pt', bin_pt, ...
      |     'arith_type', arith_type);
      settings: AttributesFormatString=slice width=8, bin_pt=7
  syncOut1 : Outport
  syncOut2 : Outport  Port=2
  dataOut : Outport  Port=3
  wires:
  syncIn/1 -> pfb_fir_real/1(sync), pfb_fir_real1/1(sync)
  uncram/1(Out1) -> pfb_fir_real/2(pol1_in1)
  uncram/2(Out2) -> pfb_fir_real/3(pol1_in2)
  uncram/3(Out3) -> pfb_fir_real/4(pol1_in3)
  uncram/4(Out4) -> pfb_fir_real/5(pol1_in4)
  uncram/5(Out5) -> pfb_fir_real1/2(pol1_in1)
  uncram/6(Out6) -> pfb_fir_real1/3(pol1_in2)
  uncram/7(Out7) -> pfb_fir_real1/4(pol1_in3)
  uncram/8(Out8) -> pfb_fir_real1/5(pol1_in4)
  pfb_fir_real/1(sync_out) -> syncOut1/1
  dataIn/1 -> uncram/1(In)
  pfb_fir_real1/1(sync_out) -> syncOut2/1
  pfb_fir_real/2(pol1_out1) -> cram/1(In1)
  pfb_fir_real/3(pol1_out2) -> cram/2(In2)
  pfb_fir_real/4(pol1_out3) -> cram/3(In3)
  pfb_fir_real/5(pol1_out4) -> cram/4(In4)
  pfb_fir_real1/2(pol1_out1) -> cram/5(In5)
  pfb_fir_real1/3(pol1_out2) -> cram/6(In6)
  pfb_fir_real1/4(pol1_out3) -> cram/7(In7)
  pfb_fir_real1/5(pol1_out4) -> cram/8(In8)
  cram/1(Out) -> dataOut/1

== system dual500MHzPFB/cfgspec/SuperSlice ==
  In : Inport  Port=1  LatchInput=off
  Slice1 : xbsIndex_r3/Slice  mode=Lower Bit Location + Width  nbits=16  bit1=-3  base1=MSB of Input  bit0=16  base0=LSB of Input  boolean_output=off  explicit_period=off  period=1  dbl_ovrd=off
  Slice10 : xbsIndex_r3/Slice  mode=Lower Bit Location + Width  nbits=1  bit1=0  base1=MSB of Input  bit0=0  base0=LSB of Input  boolean_output=on  explicit_period=off  period=1  dbl_ovrd=off
  Slice2 : xbsIndex_r3/Slice  mode=Lower Bit Location + Width  nbits=8  bit1=-2  base1=MSB of Input  bit0=8  base0=LSB of Input  boolean_output=off  explicit_period=off  period=1  dbl_ovrd=off
  Slice3 : xbsIndex_r3/Slice  mode=Lower Bit Location + Width  nbits=1  bit1=-1  base1=MSB of Input  bit0=7  base0=LSB of Input  boolean_output=on  explicit_period=off  period=1  dbl_ovrd=off
  Slice4 : xbsIndex_r3/Slice  mode=Lower Bit Location + Width  nbits=1  bit1=0  base1=MSB of Input  bit0=6  base0=LSB of Input  boolean_output=on  explicit_period=off  period=1  dbl_ovrd=off
  Slice5 : xbsIndex_r3/Slice  mode=Lower Bit Location + Width  nbits=1  bit1=0  base1=MSB of Input  bit0=5  base0=LSB of Input  boolean_output=on  explicit_period=off  period=1  dbl_ovrd=off
  Slice6 : xbsIndex_r3/Slice  mode=Lower Bit Location + Width  nbits=1  bit1=0  base1=MSB of Input  bit0=4  base0=LSB of Input  boolean_output=on  explicit_period=off  period=1  dbl_ovrd=off
  Slice7 : xbsIndex_r3/Slice  mode=Lower Bit Location + Width  nbits=1  bit1=0  base1=MSB of Input  bit0=3  base0=LSB of Input  boolean_output=on  explicit_period=off  period=1  dbl_ovrd=off
  Slice8 : xbsIndex_r3/Slice  mode=Lower Bit Location + Width  nbits=1  bit1=0  base1=MSB of Input  bit0=2  base0=LSB of Input  boolean_output=on  explicit_period=off  period=1  dbl_ovrd=off
  Slice9 : xbsIndex_r3/Slice  mode=Lower Bit Location + Width  nbits=1  bit1=0  base1=MSB of Input  bit0=1  base0=LSB of Input  boolean_output=on  explicit_period=off  period=1  dbl_ovrd=off
  "[31:16]" : Outport
  "[15:8]" : Outport  Port=2
  "[7]" : Outport  Port=3
  "[6]" : Outport  Port=4
  "[5]" : Outport  Port=5
  "[4]" : Outport  Port=6
  "[3]" : Outport  Port=7
  "[2]" : Outport  Port=8
  "[1]" : Outport  Port=9
  "[0]" : Outport  Port=10
  wires:
  In/1 -> Slice10/1, Slice9/1, Slice8/1, Slice7/1, Slice6/1, Slice5/1, Slice4/1, Slice3/1, Slice2/1, Slice1/1
  Slice1/1 -> "[31:16]"/1
  Slice2/1 -> "[15:8]"/1
  Slice3/1 -> "[7]"/1
  Slice4/1 -> "[6]"/1
  Slice5/1 -> "[5]"/1
  Slice6/1 -> "[4]"/1
  Slice7/1 -> "[3]"/1
  Slice8/1 -> "[2]"/1
  Slice9/1 -> "[1]"/1
  Slice10/1 -> "[0]"/1

== system dual500MHzPFB/cfgspec/cram ==
  In1 : Inport  Port=1  LatchInput=off
  In2 : Inport  Port=2  LatchInput=off
  In3 : Inport  Port=3  LatchInput=off
  In4 : Inport  Port=4  LatchInput=off
  Concat : S-Function  AncestorBlock=xbsIndex_r3/Concat  FunctionName=xlconcat  Parameters=sfcn_mwsv__  mask(Xilinx Bus Concatenator){num_inputs=4, explicit_period=off, period=1, dbl_ovrd=off}
      mask prompts: num_inputs "Number of Inputs"; explicit_period "Use Explicit Sample Period"; period "Sample Period  (use -1 to inherit first known input period)"; dbl_ovrd "Override with Doubles"
      mask help: Concatenates two or more inputs. Inputs must be unsigned with binary point at zero.
      mask init: same as dual500MHzPFB/cram/Concat
      mask Help: eval('xlWeb(xlhtmldoclink(''Concat''))');
      mask StyleString: popup(2|3|4|5|6|7|8|9|10|11|12|13|14|15|16),checkbox,edit,checkbox
      mask CallbackString: |xlMagicCallback||
      mask Display:
      | patch([0 iWidth iWidth 0],[0 0 iHeight iHeight] , bg);
      | patch(logoX,logoY, fg);
      | port_label('input',1,'hi');
      | port_label('input',num_inputs+1,'lo');
      | port_label('output',1,'cat');
      | ;plot([0 0 iWidth iWidth 0], [0 iHeight iHeight 0 0]);
  Reinterp{1..4} (4 alike) : xbsIndex_r3/Reinterpret  force_arith_type=on  arith_type=Unsigned  force_bin_pt=on  bin_pt=0  force_valid=on
  Out : Outport
  wires:
  Concat/1 -> Out/1
  In1/1 -> Reinterp1/1
  Reinterp1/1 -> Concat/1
  In2/1 -> Reinterp2/1
  Reinterp2/1 -> Concat/2
  In3/1 -> Reinterp3/1
  Reinterp3/1 -> Concat/3
  In4/1 -> Reinterp4/1
  Reinterp4/1 -> Concat/4

== system dual500MHzPFB/cfgspec/cram1 ==
  In1 : Inport  Port=1  LatchInput=off
  In2 : Inport  Port=2  LatchInput=off
  In3 : Inport  Port=3  LatchInput=off
  In4 : Inport  Port=4  LatchInput=off
  In5 : Inport  Port=5  LatchInput=off
  In6 : Inport  Port=6  LatchInput=off
  In7 : Inport  Port=7  LatchInput=off
  In8 : Inport  Port=8  LatchInput=off
  Concat : S-Function  AncestorBlock=xbsIndex_r3/Concat  FunctionName=xlconcat  Parameters=sfcn_mwsv__  mask(Xilinx Bus Concatenator){num_inputs=8, explicit_period=off, period=1, dbl_ovrd=off}
      mask prompts: num_inputs "Number of Inputs"; explicit_period "Use Explicit Sample Period"; period "Sample Period  (use -1 to inherit first known input period)"; dbl_ovrd "Override with Doubles"
      mask help: Concatenates two or more inputs. Inputs must be unsigned with binary point at zero.
      mask init: same as dual500MHzPFB/cram/Concat
      mask Help: eval('xlWeb(xlhtmldoclink(''Concat''))');
      mask StyleString: popup(2|3|4|5|6|7|8|9|10|11|12|13|14|15|16),checkbox,edit,checkbox
      mask CallbackString: |xlMagicCallback||
      mask Display:
      | patch([0 iWidth iWidth 0],[0 0 iHeight iHeight] , bg);
      | patch(logoX,logoY, fg);
      | port_label('input',1,'hi');
      | port_label('input',num_inputs+1,'lo');
      | port_label('output',1,'cat');
      | ;plot([0 0 iWidth iWidth 0], [0 iHeight iHeight 0 0]);
  Reinterp{1..8} (8 alike) : xbsIndex_r3/Reinterpret  force_arith_type=on  arith_type=Unsigned  force_bin_pt=on  bin_pt=0  force_valid=on
  Out : Outport
  wires:
  Concat/1 -> Out/1
  In1/1 -> Reinterp1/1
  Reinterp1/1 -> Concat/1
  In2/1 -> Reinterp2/1
  Reinterp2/1 -> Concat/2
  In3/1 -> Reinterp3/1
  Reinterp3/1 -> Concat/3
  In4/1 -> Reinterp4/1
  Reinterp4/1 -> Concat/4
  In5/1 -> Reinterp5/1
  Reinterp5/1 -> Concat/5
  In6/1 -> Reinterp6/1
  Reinterp6/1 -> Concat/6
  In7/1 -> Reinterp7/1
  Reinterp7/1 -> Concat/7
  In8/1 -> Reinterp8/1
  Reinterp8/1 -> Concat/8

== system dual500MHzPFB/cfgspec/nCasts1 ==
  In1 : Inport  Port=1  LatchInput=off
  In2 : Inport  Port=2  LatchInput=off
  In3 : Inport  Port=3  LatchInput=off
  In4 : Inport  Port=4  LatchInput=off
  Cast{1..4} (4 alike) : xbsIndex_r3/Convert  arith_type=Unsigned  n_bits=32  bin_pt=31  quantization=Truncate  overflow=Wrap  latency=0  explicit_period=off  period=1  dbl_ovrd=off  show_param=off  inserted_by_tool=off  pipeline=off
      settings: xl_area=[0, 0, 0, 0, 0, 0, 0]
  Out1 : Outport
  Out2 : Outport  Port=2
  Out3 : Outport  Port=3
  Out4 : Outport  Port=4
  wires:
  In1/1 -> Cast1/1
  Cast1/1 -> Out1/1
  In2/1 -> Cast2/1
  Cast2/1 -> Out2/1
  In3/1 -> Cast3/1
  Cast3/1 -> Out3/1
  In4/1 -> Cast4/1
  Cast4/1 -> Out4/1

== system dual500MHzPFB/cfgspec/power ==
  c : Inport  Port=1  LatchInput=off
  c_to_ri : casper_library/Misc/c_to_ri  n_bits=BitWidth  bin_pt=BitWidth-1
      settings: AttributesFormatString=18_17 r/i
  imag_square : xbsIndex_r3/Mult  precision=Full  arith_type="Signed  (2's comp)"  n_bits=8  bin_pt=2  quantization=Truncate  overflow=Wrap  latency=mult_latency  explicit_period=off  period=1  en=off  dbl_ovrd=off  show_param=on  mult_type=Parallel  oversample=2  use_embedded=on  pipeline=on  use_rpm=on  placement_style=Rectangular Shape  gen_core=off
      settings: xl_area=[0, 0, 0, 0, 0, 0, 0]
  power_adder : xbsIndex_r3/AddSub  mode=Addition  precision=User Defined  arith_type=Unsigned  n_bits=BitWidth * 2  bin_pt=BitWidth * 2 - 1  quantization=Truncate  overflow=Wrap  latency=add_latency  explicit_period=off  period=1  use_carryin=off  use_carryout=off  en=off  dbl_ovrd=off  show_param=on  use_core=on  pipeline=on  use_rpm=on  gen_core=off
      settings: xl_area=[0, 0, 0, 0, 0, 0, 0]
  real_square : xbsIndex_r3/Mult  precision=Full  arith_type="Signed  (2's comp)"  n_bits=8  bin_pt=2  quantization=Truncate  overflow=Wrap  latency=mult_latency  explicit_period=off  period=1  en=off  dbl_ovrd=off  show_param=on  mult_type=Parallel  oversample=2  use_embedded=on  pipeline=on  use_rpm=on  placement_style=Rectangular Shape  gen_core=off
      settings: xl_area=[0, 0, 0, 0, 0, 0, 0]
  power : Outport
  wires:
  power_adder/1 -> power/1
  imag_square/1 -> power_adder/2
  real_square/1 -> power_adder/1
  c/1 -> c_to_ri/1
  c_to_ri/1 -> real_square/1, real_square/2
  c_to_ri/2 -> imag_square/2, imag_square/1

== system dual500MHzPFB/cfgspec/power1 ==
  c : Inport  Port=1  LatchInput=off
  c_to_ri : casper_library/Misc/c_to_ri  n_bits=BitWidth  bin_pt=BitWidth-1
      settings: AttributesFormatString=18_17 r/i
  imag_square : xbsIndex_r3/Mult  precision=Full  arith_type="Signed  (2's comp)"  n_bits=8  bin_pt=2  quantization=Truncate  overflow=Wrap  latency=mult_latency  explicit_period=off  period=1  en=off  dbl_ovrd=off  show_param=on  mult_type=Parallel  oversample=2  use_embedded=on  pipeline=on  use_rpm=on  placement_style=Rectangular Shape  gen_core=off
      settings: xl_area=[0, 0, 0, 0, 0, 0, 0]
  power_adder : xbsIndex_r3/AddSub  mode=Addition  precision=User Defined  arith_type=Unsigned  n_bits=BitWidth * 2  bin_pt=BitWidth * 2 - 1  quantization=Truncate  overflow=Wrap  latency=add_latency  explicit_period=off  period=1  use_carryin=off  use_carryout=off  en=off  dbl_ovrd=off  show_param=on  use_core=on  pipeline=on  use_rpm=on  gen_core=off
      settings: xl_area=[0, 0, 0, 0, 0, 0, 0]
  real_square : xbsIndex_r3/Mult  precision=Full  arith_type="Signed  (2's comp)"  n_bits=8  bin_pt=2  quantization=Truncate  overflow=Wrap  latency=mult_latency  explicit_period=off  period=1  en=off  dbl_ovrd=off  show_param=on  mult_type=Parallel  oversample=2  use_embedded=on  pipeline=on  use_rpm=on  placement_style=Rectangular Shape  gen_core=off
      settings: xl_area=[0, 0, 0, 0, 0, 0, 0]
  power : Outport
  wires:
  c_to_ri/2 -> imag_square/1, imag_square/2
  c_to_ri/1 -> real_square/2, real_square/1
  c/1 -> c_to_ri/1
  real_square/1 -> power_adder/1
  imag_square/1 -> power_adder/2
  power_adder/1 -> power/1
